simulink model "gm_transmitter"  (R2020b)
settings: Solver=FixedStepDiscrete  StartTime=0.0  StopTime=30  RelTol=1e-3
libraries: dspsigops x3, dspmlti4 x2, hdlmdlgenlib x2, commrandsrc3 x1
settings Model: Creator=wardo  LastModifiedBy=wardo
settings DataIOCC: LimitDataPoints=on  SaveOutput=off  SaveTime=off
settings OptimizationCC: BlockReduction=off  ConditionallyExecuteInputs=off  DefaultParameterBehavior=Inlined  LifeSpan=inf
settings DebuggingCC: AlgebraicLoopMsg=error  InheritedTsInSrcMsg=none  SingleTaskRateTransMsg=error  AllowSymbolicDim=off  StrictBusMsg=ErrorOnBusTreatedAsVector  SFUnexpectedBacktrackingDiag=warning  SFNoUnconditionalDefaultTransitionDiag=warning  SFExecutionAtInitializationDiag=none  ArithmeticOperatorsInVariantConditions=warning
settings HardwareCC: ProdBitPerPointer=32  ProdBitPerSizeT=32  ProdBitPerPtrDiffT=32  ProdLargestAtomicFloat=None  ProdIntDivRoundTo=Undefined  ProdEndianess=Unspecified  ProdWordSize=32  ProdHWDeviceType=ASIC/FPGA->ASIC/FPGA  ProdEqTarget=off
settings SFSimCC: SimUseLocalCustomCode=off  CustomCodeUndefinedFunction=UseInterfaceOnly
settings RTWCC: RTWUseLocalCustomCode=off
settings CodeAppCC: StateflowObjectComments=on
settings GRTTargetCC: TargetLangStandard=C89/C90 (ANSI)
settings ConfigComp: CovScope=ReferencedModels  CovMetricSettings=dw  CovSaveCumulativeToWorkspaceVar=on  CovSaveSingleToWorkspaceVar=on  CovExternalEMLEnable=off  CovSFcnEnable=off

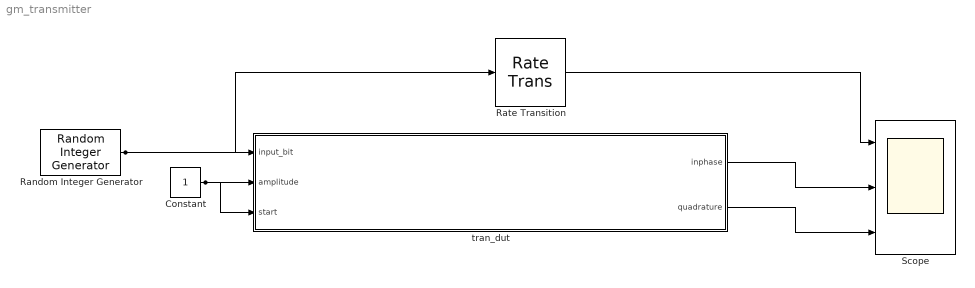
== system gm_transmitter ==
  Constant : Constant  OutDataTypeStr=uint8  SampleTime=-1
  Random Integer Generator : commrandsrc3/Random Integer Generator  SetSize=2  SeedSource=Auto  Seed=0  SampleTime=1  SamplesPerFrame=1  OutputDataType=boolean  SimulateUsing=Code generation
  Rate Transition : RateTransition
  Scope : Scope  NumInputPorts=3
  tran_dut : Subsystem
  wires:
  Rate Transition/1 -> Scope/1
  Constant/1 -> tran_dut/2(amplitude), tran_dut/3(start)
  tran_dut/1(inphase) -> Scope/2
  tran_dut/2(quadrature) -> Scope/3
  Random Integer Generator/1 -> tran_dut/1(input_bit), Rate Transition/1

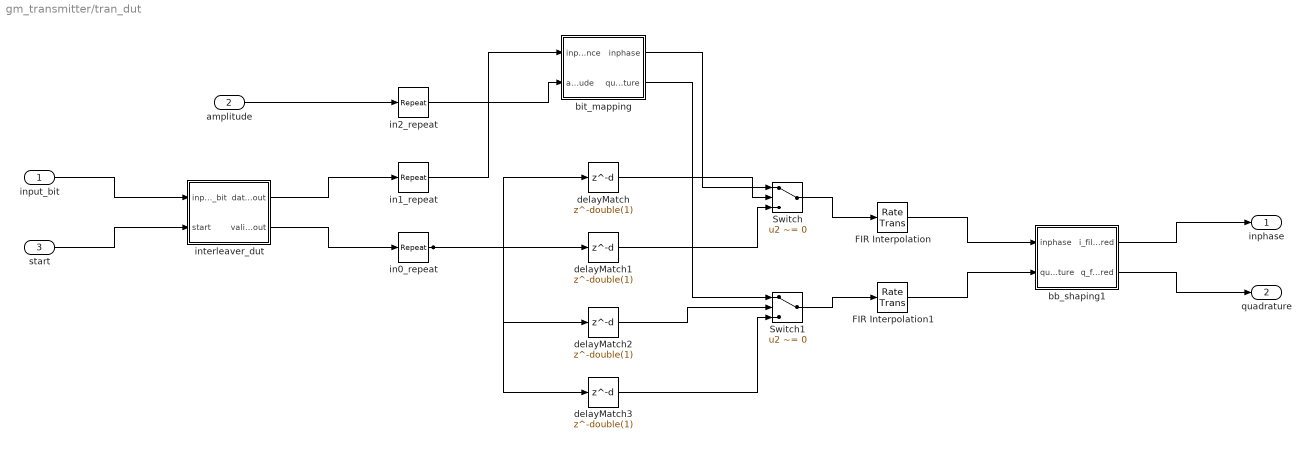
== system gm_transmitter/tran_dut ==
  input_bit : Inport  OutDataTypeStr=boolean  PortDimensions=1  SampleTime=1
  amplitude : Inport  Port=2  OutDataTypeStr=uint8  PortDimensions=1  SampleTime=1
  start : Inport  Port=3  OutDataTypeStr=uint8  PortDimensions=1  SampleTime=1
  FIR Interpolation : RateTransition  OutPortSampleTimeOpt=Multiple of input port sample time  OutPortSampleTimeMultiple=8
  FIR Interpolation1 : RateTransition  OutPortSampleTimeOpt=Multiple of input port sample time  OutPortSampleTimeMultiple=8
  Switch : Switch  Criteria=u2 ~= 0  Threshold=double(0)  OutDataTypeStr=fixdt(1, 25, 15)  SampleTime=0.125
  Switch1 : Switch  Criteria=u2 ~= 0  Threshold=double(0)  OutDataTypeStr=fixdt(1, 25, 15)  SampleTime=0.125
  bb_shaping1 : Subsystem
  bit_mapping : Subsystem
  delayMatch{,1..3} (4 alike) : Delay  DelayLength=double(1)  InitialCondition=0  SampleTime=0.125
  in0_repeat : dspsigops/Repeat  N=double(8)  RateOptions=Allow multirate processing  ic=0  mode=Unused parameter value
  in1_repeat : dspsigops/Repeat  N=double(8)  RateOptions=Allow multirate processing  ic=0  mode=Unused parameter value
  in2_repeat : dspsigops/Repeat  N=double(8)  RateOptions=Allow multirate processing  ic=0  mode=Unused parameter value
  interleaver_dut : Subsystem
  inphase : Outport  VectorParamsAs1DForOutWhenUnconnected=off
  quadrature : Outport  Port=2  VectorParamsAs1DForOutWhenUnconnected=off
  wires:
  input_bit/1 -> interleaver_dut/1(input_bit)
  amplitude/1 -> in2_repeat/1
  start/1 -> interleaver_dut/2(start)
  bb_shaping1/1(i_filtered) -> inphase/1
  bb_shaping1/2(q_filtered) -> quadrature/1
  interleaver_dut/1(data_out) -> in1_repeat/1
  interleaver_dut/2(valid_out) -> in0_repeat/1
  FIR Interpolation/1 -> bb_shaping1/1(inphase)
  FIR Interpolation1/1 -> bb_shaping1/2(quadrature)
  Switch/1 -> FIR Interpolation/1
  Switch1/1 -> FIR Interpolation1/1
  in0_repeat/1 -> delayMatch3/1, delayMatch2/1, delayMatch1/1, delayMatch/1
  in1_repeat/1 -> bit_mapping/1(input_sequence)
  in2_repeat/1 -> bit_mapping/2(amplitude)
  bit_mapping/1(inphase) -> Switch/1
  bit_mapping/2(quadrature) -> Switch1/1
  delayMatch/1 -> Switch/2
  delayMatch1/1 -> Switch/3
  delayMatch2/1 -> Switch1/2
  delayMatch3/1 -> Switch1/3

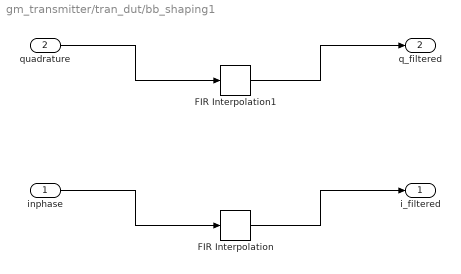
== system gm_transmitter/tran_dut/bb_shaping1 ==
  inphase : Inport  OutDataTypeStr=fixdt(1, 25, 15)  PortDimensions=1  SampleTime=1
  quadrature : Inport  Port=2  OutDataTypeStr=fixdt(1, 25, 15)  PortDimensions=1  SampleTime=1
  FIR Interpolation : dspmlti4/FIR Interpolation  FilterSource=Dialog parameters  PrivateCoeffs=0  h=[-0.00599670410156250,-0.00514221191406250,-0.00289916992187500,0.000442504882812500,0.00431823730468750,0.00794982910156250,0.0104980468750000,0.0112304687500000,0.00967407226562500,0.00578308105468750,0,-0.00680541992187500,-0.0134124755859375,-0.0184326171875000,-0.0205841064453125,-0.0189819335937500,-0.0133361816406250,-0.00410461425781250,0.00752258300781250,0.0196380615234375,0.0300140380859375,0.0363464355468750,0.0367584228515625,0.0301208496093750,0.0164794921875000,-0.00291442871093750,-0.0254821777343750,-0.0476837158203125,-0.0653228759765625,-0.0742187500000000,-0.0707244873046875,-0.0524291992187500,-0.0185852050781250,0.0296783447265625,0.0892028808593750,0.155227661132813,0.221755981445313,0.282333374023438,0.330810546875000,0.362121582031250,0.372940063476563,0.362121582031250,0.330810546875000,0.282333374023438,0.221755981445313,0.155227661132813,0.0892028808593750,0.0296783447265625,-0.0185852050781250,-0.0524291992187500,-0.0707244873046875,-0.0742187500000000,-0.0653228759765625,-0.0476837158203125,-0.0254821777343750,-0.00291442871093750,0.0164794921875000,0.0301208496093750,0.0367584228515625,0.0363464355468750,0.0300140380859375,0.0196380615234375,0.00752258300781250,-0.00410461425781250,-0.0133361816406250,-0.0189819335937500,-0.0205841064453125,-0.0184326171875000,-0.0134124755859375,-0.00680541992187500,0,0.00578308105468750,0.00967407226562500,0.0112304687500000,0.0104980468750000,0.00794982910156250,0.00431823730468750,0.000442504882812500,-0.00289916992187500,-0.00514221191406250,-0.00599670410156250]  L=8  FilterObject=FINTERP  framing=Allow multirate processing  outputBufInitCond=0  roundingMode=Floor  overflowMode=off  firstCoeffMode=Specify word length  firstCoeffWordLength=16  firstCoeffFracLength=15  firstCoeffDataTypeStr=fixdt(1,16)  firstCoeffMin=[]  firstCoeffMax=[]  firstCoeffLastDataTypeStr=fixdt(1,16)  outputDataTypeStr=Inherit: Same as accumulator  outputMin=[]  outputMax=[]  outputLastDataTypeStr=Inherit: Same as accumulator
      settings: SourceProductName=DSP System Toolbox
  FIR Interpolation1 : dspmlti4/FIR Interpolation  FilterSource=Dialog parameters  PrivateCoeffs=0  h=[-0.00599670410156250,-0.00514221191406250,-0.00289916992187500,0.000442504882812500,0.00431823730468750,0.00794982910156250,0.0104980468750000,0.0112304687500000,0.00967407226562500,0.00578308105468750,0,-0.00680541992187500,-0.0134124755859375,-0.0184326171875000,-0.0205841064453125,-0.0189819335937500,-0.0133361816406250,-0.00410461425781250,0.00752258300781250,0.0196380615234375,0.0300140380859375,0.0363464355468750,0.0367584228515625,0.0301208496093750,0.0164794921875000,-0.00291442871093750,-0.0254821777343750,-0.0476837158203125,-0.0653228759765625,-0.0742187500000000,-0.0707244873046875,-0.0524291992187500,-0.0185852050781250,0.0296783447265625,0.0892028808593750,0.155227661132813,0.221755981445313,0.282333374023438,0.330810546875000,0.362121582031250,0.372940063476563,0.362121582031250,0.330810546875000,0.282333374023438,0.221755981445313,0.155227661132813,0.0892028808593750,0.0296783447265625,-0.0185852050781250,-0.0524291992187500,-0.0707244873046875,-0.0742187500000000,-0.0653228759765625,-0.0476837158203125,-0.0254821777343750,-0.00291442871093750,0.0164794921875000,0.0301208496093750,0.0367584228515625,0.0363464355468750,0.0300140380859375,0.0196380615234375,0.00752258300781250,-0.00410461425781250,-0.0133361816406250,-0.0189819335937500,-0.0205841064453125,-0.0184326171875000,-0.0134124755859375,-0.00680541992187500,0,0.00578308105468750,0.00967407226562500,0.0112304687500000,0.0104980468750000,0.00794982910156250,0.00431823730468750,0.000442504882812500,-0.00289916992187500,-0.00514221191406250,-0.00599670410156250]  L=8  FilterObject=FINTERP  framing=Allow multirate processing  outputBufInitCond=0  roundingMode=Floor  overflowMode=off  firstCoeffMode=Specify word length  firstCoeffWordLength=16  firstCoeffFracLength=15  firstCoeffDataTypeStr=fixdt(1,16)  firstCoeffMin=[]  firstCoeffMax=[]  firstCoeffLastDataTypeStr=fixdt(1,16)  outputDataTypeStr=Inherit: Same as accumulator  outputMin=[]  outputMax=[]  outputLastDataTypeStr=Inherit: Same as accumulator
      settings: SourceProductName=DSP System Toolbox
  i_filtered : Outport  VectorParamsAs1DForOutWhenUnconnected=off
  q_filtered : Outport  Port=2  VectorParamsAs1DForOutWhenUnconnected=off
  wires:
  FIR Interpolation/1 -> i_filtered/1
  FIR Interpolation1/1 -> q_filtered/1
  inphase/1 -> FIR Interpolation/1
  quadrature/1 -> FIR Interpolation1/1

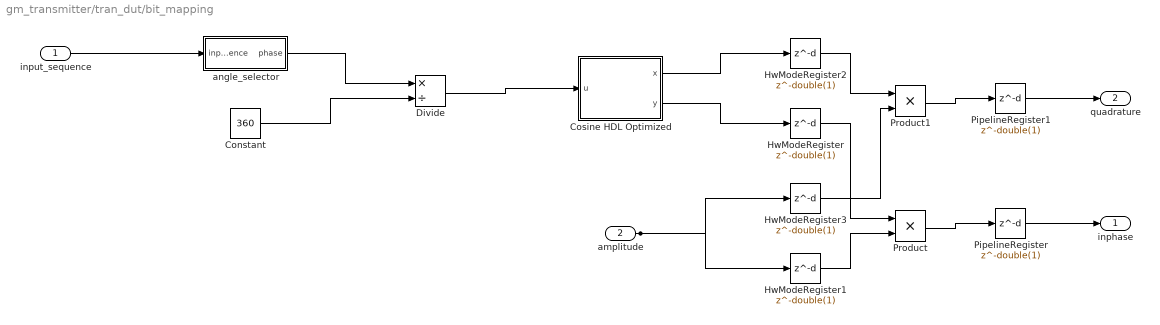
== system gm_transmitter/tran_dut/bit_mapping ==
  input_sequence : Inport  OutDataTypeStr=fixdt(0, 1, 0)  PortDimensions=[1 3]  SampleTime=0.125
  amplitude : Inport  Port=2  OutDataTypeStr=uint8  PortDimensions=1  SampleTime=0.125
  Constant : Constant  Value=360  OutDataTypeStr=fixdt(0, 9, 0)  SampleTime=0.125
  Cosine HDL Optimized : Subsystem  mask(Sine and Cosine HDL optimized block){OutputFormula=sin(2*pi*u) and cos(2*pi*u), NumDataPoints=double(64), TableDataTypeStr=fixdt(1,16,15), SimulateLUTROMDelay=off}
      mask prompts: OutputFormula "Simulink:masks:OutputFormula_MP"; NumDataPoints "HDLShared:hdlshared:CosineHDL_Npts"; TableDataTypeStr "Simulink:blkprm_prompts:TABLE_UNIFIEDDATATYPE"; SimulateLUTROMDelay "HDLShared:hdlshared:CosineHDL_Map2RAM"
      mask help: Sine and Cosine HDL optimized block using quarter wave symmetry, and HDL friendly settings.
      mask Help: helpview([docroot '/hdlcoder/helptargets.map'],'SineAndCosineHDL_Optimized');
      mask TypeOptions OutputFormula: sin(2*pi*u) | cos(2*pi*u) | exp(j*2*pi*u) | sin(2*pi*u) and cos(2*pi*u)
      mask Display:
      | port_label('input',1,'u')
      | port_label('output',1,'sin(2*pi*u)')
      | port_label('output',2,'cos(2*pi*u)')
      | xpos = 0.35;
      | yoffset = 0.5;
      | if ( SimulateLUTROMDelay )
      |   text(xpos,yoffset,'HDL (Z^{-1})','texmode','on')
      | else
      |    text(xpos,yoffset,'HDL')
      | end
  Divide : Product  Inputs=*/  OutDataTypeStr=fixdt(1, 16, 14)  RndMeth=Zero  SaturateOnIntegerOverflow=on  SampleTime=0.125
  HwModeRegister{,1..3} (4 alike) : Delay  DelayLength=double(1)  InitialCondition=0  SampleTime=0.125
  PipelineRegister : Delay  DelayLength=double(1)  InitialCondition=0  SampleTime=0.125
  PipelineRegister1 : Delay  DelayLength=double(1)  InitialCondition=0  SampleTime=0.125
  Product : Product  Inputs=**  OutDataTypeStr=fixdt(1, 25, 15)  SampleTime=0.125
  Product1 : Product  Inputs=**  OutDataTypeStr=fixdt(1, 25, 15)  SampleTime=0.125
  angle_selector : Subsystem
  inphase : Outport  VectorParamsAs1DForOutWhenUnconnected=off
  quadrature : Outport  Port=2  VectorParamsAs1DForOutWhenUnconnected=off
  wires:
  Constant/1 -> Divide/2
  Cosine HDL Optimized/1(x) -> HwModeRegister2/1
  Cosine HDL Optimized/2(y) -> HwModeRegister/1
  Divide/1 -> Cosine HDL Optimized/1(u)
  PipelineRegister/1 -> inphase/1
  PipelineRegister1/1 -> quadrature/1
  angle_selector/1(phase) -> Divide/1
  input_sequence/1 -> angle_selector/1(input_sequence)
  amplitude/1 -> HwModeRegister1/1, HwModeRegister3/1
  Product/1 -> PipelineRegister/1
  HwModeRegister/1 -> Product/1
  HwModeRegister1/1 -> Product/2
  Product1/1 -> PipelineRegister1/1
  HwModeRegister2/1 -> Product1/1
  HwModeRegister3/1 -> Product1/2

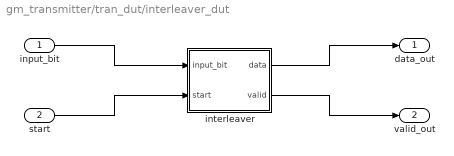
== system gm_transmitter/tran_dut/interleaver_dut ==
  input_bit : Inport  OutDataTypeStr=boolean  PortDimensions=1  SampleTime=1
  start : Inport  Port=2  OutDataTypeStr=uint8  PortDimensions=1  SampleTime=1
  interleaver : Subsystem
  data_out : Outport  VectorParamsAs1DForOutWhenUnconnected=off
  valid_out : Outport  Port=2  VectorParamsAs1DForOutWhenUnconnected=off
  wires:
  interleaver/1(data) -> data_out/1
  interleaver/2(valid) -> valid_out/1
  input_bit/1 -> interleaver/1(input_bit)
  start/1 -> interleaver/2(start)

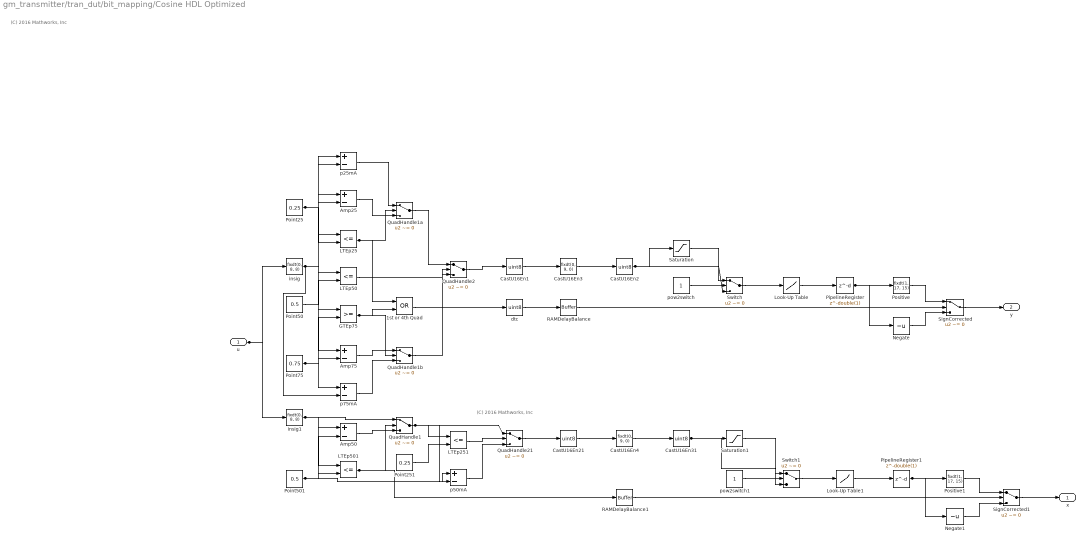
== system gm_transmitter/tran_dut/bit_mapping/Cosine HDL Optimized ==
  note: (C) 2016 Mathworks, Inc
  note: (C) 2016 Mathworks, Inc
  u : Inport  OutDataTypeStr=fixdt(1, 16, 14)  SampleTime=0.125
  1st or 4th Quad : Logic  Operator=OR  AllPortsSameDT=off  OutDataTypeStr=boolean  SampleTime=0.125
  Amp25 : Sum  Inputs=+-  AccumDataTypeStr=fixdt(1, 18, 17)  OutDataTypeStr=fixdt(1, 18, 17)  SampleTime=0.125
  Amp50 : Sum  Inputs=+-  AccumDataTypeStr=fixdt(1, 18, 17)  OutDataTypeStr=fixdt(1, 18, 17)  SampleTime=0.125
  Amp75 : Sum  Inputs=+-  AccumDataTypeStr=fixdt(1, 18, 17)  OutDataTypeStr=fixdt(1, 18, 17)  SampleTime=0.125
  CastU16En1 : DataTypeConversion  OutDataTypeStr=uint8  ConvertRealWorld=Stored Integer (SI)  SampleTime=0.125
  CastU16En2 : DataTypeConversion  OutDataTypeStr=uint8  ConvertRealWorld=Stored Integer (SI)  SampleTime=0.125  SaturateOnIntegerOverflow=on
  CastU16En21 : DataTypeConversion  OutDataTypeStr=uint8  ConvertRealWorld=Stored Integer (SI)  SampleTime=0.125
  CastU16En3 : DataTypeConversion  OutDataTypeStr=fixdt(0, 9, 0)  SampleTime=0.125
  CastU16En31 : DataTypeConversion  OutDataTypeStr=uint8  ConvertRealWorld=Stored Integer (SI)  SampleTime=0.125  SaturateOnIntegerOverflow=on
  CastU16En4 : DataTypeConversion  OutDataTypeStr=fixdt(0, 9, 0)  SampleTime=0.125
  GTEp75 : RelationalOperator  OutDataTypeStr=boolean  SampleTime=0.125  RndMeth=Nearest
  LTEp{25,50,251,501} (4 alike) : RelationalOperator  Operator=<=  OutDataTypeStr=boolean  SampleTime=0.125  RndMeth=Nearest
  Look-Up Table : Lookup_n-D  NumberOfTableDimensions=1  BreakpointsForDimension1="fi(\"numerictype\",numerictype(0,8,0),\"fimath\",fimath(\"RoundingMethod\", \"Floor\",\"OverflowAction\", \"Wrap\",\"ProductMode\",\"FullPrecision\",\"SumMode\",\"FullPrecision\"),\"Value\",\"[0 1 2 3 4 5 6 7 8 9 10 11 12 13 14 15 16 17 18 19 20 21 22 23 24 25 26 27 28 29 30 31 32 33 34 35 36 37 38 39 40 41 42 43 44 45 46 47 48 49 50 51 52 53 54 55 56 57 58 59 60 61 62 63]\")"  Table="reshape(fi(\"numerictype\",numerictype(1,17,15),\"fimath\",fimath(\"RoundingMethod\", \"Floor\",\"OverflowAction\", \"Wrap\",\"ProductMode\",\"FullPrecision\",\"SumMode\",\"FullPrecision\"),\"Value\",\"[0;0.024932861328125;0.049835205078125;0.074737548828125;0.099578857421875;0.12432861328125;0.1490478515625;0.17364501953125;0.198150634765625;0.2225341796875;0.24676513671875;0.270843505859375;0.294769287109375;0.3184814453125;0.342010498046875;0.365325927734375;0.388427734375;0.411285400390625;0.43389892578125;0.456207275390625;0.478240966796875;0.5;0.52142333984375;0.54254150390625;0.563323974609375;0.583740234375;0.603790283203125;0.623504638671875;0.642791748046875;0.66168212890625;0.68017578125;0.6982421875;0.71588134765625;0.733062744140625;0.749786376953125;0.76605224609375;0.781829833984375;0.797119140625;0.81195068359375;0.82623291015625;0.84002685546875;0.853302001953125;0.86602783203125;0.87823486328125;0.889862060546875;0.900970458984375;0.9114990234375;0.921478271484375;0.930877685546875;0.939697265625;0.94793701171875;0.95556640625;0.962615966796875;0.969085693359375;0.97491455078125;0.98016357421875;0.98480224609375;0.98883056640625;0.99224853515625;0.995025634765625;0.9971923828125;0.998748779296875;0.99969482421875;1]\"), [1  64])"  InterpMethod=Flat  ExtrapMethod=Clip  DiagnosticForOutOfRangeInput=Error  SampleTime=0.125  OutDataTypeStr=fixdt(1, 17, 15)  InputSameDT=on
  Look-Up Table1 : Lookup_n-D  NumberOfTableDimensions=1  BreakpointsForDimension1="fi(\"numerictype\",numerictype(0,8,0),\"fimath\",fimath(\"RoundingMethod\", \"Floor\",\"OverflowAction\", \"Wrap\",\"ProductMode\",\"FullPrecision\",\"SumMode\",\"FullPrecision\"),\"Value\",\"[0 1 2 3 4 5 6 7 8 9 10 11 12 13 14 15 16 17 18 19 20 21 22 23 24 25 26 27 28 29 30 31 32 33 34 35 36 37 38 39 40 41 42 43 44 45 46 47 48 49 50 51 52 53 54 55 56 57 58 59 60 61 62 63]\")"  Table="reshape(fi(\"numerictype\",numerictype(1,17,15),\"fimath\",fimath(\"RoundingMethod\", \"Floor\",\"OverflowAction\", \"Wrap\",\"ProductMode\",\"FullPrecision\",\"SumMode\",\"FullPrecision\"),\"Value\",\"[0;0.024932861328125;0.049835205078125;0.074737548828125;0.099578857421875;0.12432861328125;0.1490478515625;0.17364501953125;0.198150634765625;0.2225341796875;0.24676513671875;0.270843505859375;0.294769287109375;0.3184814453125;0.342010498046875;0.365325927734375;0.388427734375;0.411285400390625;0.43389892578125;0.456207275390625;0.478240966796875;0.5;0.52142333984375;0.54254150390625;0.563323974609375;0.583740234375;0.603790283203125;0.623504638671875;0.642791748046875;0.66168212890625;0.68017578125;0.6982421875;0.71588134765625;0.733062744140625;0.749786376953125;0.76605224609375;0.781829833984375;0.797119140625;0.81195068359375;0.82623291015625;0.84002685546875;0.853302001953125;0.86602783203125;0.87823486328125;0.889862060546875;0.900970458984375;0.9114990234375;0.921478271484375;0.930877685546875;0.939697265625;0.94793701171875;0.95556640625;0.962615966796875;0.969085693359375;0.97491455078125;0.98016357421875;0.98480224609375;0.98883056640625;0.99224853515625;0.995025634765625;0.9971923828125;0.998748779296875;0.99969482421875;1]\"), [1  64])"  InterpMethod=Flat  ExtrapMethod=Clip  DiagnosticForOutOfRangeInput=Error  SampleTime=0.125  OutDataTypeStr=fixdt(1, 17, 15)  InputSameDT=on
  Negate : UnaryMinus  SampleTime=0.125
  Negate1 : UnaryMinus  SampleTime=0.125
  PipelineRegister : Delay  DelayLength=double(1)  InitialCondition=0  SampleTime=0.125
  PipelineRegister1 : Delay  DelayLength=double(1)  InitialCondition=0  SampleTime=0.125
  Point25 : Constant  Value=0.25  OutDataTypeStr=fixdt(0, 17, 17)  SampleTime=0.125
  Point251 : Constant  Value=0.25  OutDataTypeStr=fixdt(0, 17, 17)  SampleTime=0.125
  Point50 : Constant  Value=0.5  OutDataTypeStr=fixdt(0, 17, 17)  SampleTime=0.125
  Point501 : Constant  Value=0.5  OutDataTypeStr=fixdt(0, 17, 17)  SampleTime=0.125
  Point75 : Constant  Value=0.75  OutDataTypeStr=fixdt(0, 17, 17)  SampleTime=0.125
  Positive : DataTypeConversion  OutDataTypeStr=fixdt(1, 17, 15)  SampleTime=0.125
  Positive1 : DataTypeConversion  OutDataTypeStr=fixdt(1, 17, 15)  SampleTime=0.125
  QuadHandle1 : Switch  Criteria=u2 ~= 0  Threshold=double(0)  OutDataTypeStr=fixdt(1, 18, 17)  SampleTime=0.125
  QuadHandle1a : Switch  Criteria=u2 ~= 0  Threshold=double(0)  OutDataTypeStr=fixdt(1, 18, 17)  SampleTime=0.125
  QuadHandle1b : Switch  Criteria=u2 ~= 0  Threshold=double(0)  OutDataTypeStr=fixdt(1, 18, 17)  SampleTime=0.125
  QuadHandle2 : Switch  Criteria=u2 ~= 0  Threshold=double(0)  OutDataTypeStr=fixdt(0, 8, 8)  SampleTime=0.125  SaturateOnIntegerOverflow=on
  QuadHandle21 : Switch  Criteria=u2 ~= 0  Threshold=double(0)  OutDataTypeStr=fixdt(0, 8, 8)  SampleTime=0.125
  RAMDelayBalance : hdlmdlgenlib/Buffer
      settings: SourceProductBaseCode=SL
  RAMDelayBalance1 : hdlmdlgenlib/Buffer
      settings: SourceProductBaseCode=SL
  Saturation : Saturate  UpperLimit="fi(0,0,8,0,\"hex\",\"3f\")"  LowerLimit="fi(0,0,8,0,\"hex\",\"00\")"  SampleTime=0.125  OutDataTypeStr=uint8
  Saturation1 : Saturate  UpperLimit="fi(0,0,8,0,\"hex\",\"3f\")"  LowerLimit="fi(0,0,8,0,\"hex\",\"00\")"  SampleTime=0.125  OutDataTypeStr=uint8
  SignCorrected : Switch  Criteria=u2 ~= 0  Threshold=double(0)  OutDataTypeStr=fixdt(1, 17, 15)  SampleTime=0.125
  SignCorrected1 : Switch  Criteria=u2 ~= 0  Threshold=double(0)  OutDataTypeStr=fixdt(1, 17, 15)  SampleTime=0.125
  Switch : Switch  Criteria=u2 ~= 0  Threshold=double(0)  OutDataTypeStr=uint8  SampleTime=0.125
  Switch1 : Switch  Criteria=u2 ~= 0  Threshold=double(0)  OutDataTypeStr=uint8  SampleTime=0.125
  dtc : DataTypeConversion  OutDataTypeStr=uint8  SampleTime=0.125
  insig : DataTypeConversion  OutDataTypeStr=fixdt(0, 8, 8)  SampleTime=0.125
  insig1 : DataTypeConversion  OutDataTypeStr=fixdt(0, 8, 8)  SampleTime=0.125
  p25mA : Sum  Inputs=+-  AccumDataTypeStr=fixdt(1, 18, 17)  OutDataTypeStr=fixdt(1, 18, 17)  SampleTime=0.125
  p50mA : Sum  Inputs=+-  AccumDataTypeStr=fixdt(1, 19, 17)  OutDataTypeStr=fixdt(1, 19, 17)  SampleTime=0.125
  p75mA : Sum  Inputs=+-  AccumDataTypeStr=fixdt(1, 18, 17)  OutDataTypeStr=fixdt(1, 18, 17)  SampleTime=0.125
  pow2switch : Constant  OutDataTypeStr=boolean  SampleTime=0.125
  pow2switch1 : Constant  OutDataTypeStr=boolean  SampleTime=0.125
  x : Outport
  y : Outport  Port=2
  wires:
  dtc/1 -> RAMDelayBalance/1
  Amp25/1 -> QuadHandle1a/3
  Amp75/1 -> QuadHandle1b/1
  CastU16En1/1 -> CastU16En3/1
  CastU16En2/1 -> Switch/3, Saturation/1
  CastU16En3/1 -> CastU16En2/1
  GTEp75/1 -> QuadHandle1b/2, 1st or 4th Quad/2
  LTEp25/1 -> QuadHandle1a/2, 1st or 4th Quad/1
  LTEp50/1 -> QuadHandle2/2
  PipelineRegister/1 -> Positive/1, Negate/1
  Negate/1 -> SignCorrected/3
  Point25/1 -> p25mA/1, LTEp25/2, Amp25/2
  Point50/1 -> LTEp50/2
  Point75/1 -> p75mA/1, GTEp75/2, Amp75/2
  Positive/1 -> SignCorrected/1
  QuadHandle1a/1 -> QuadHandle2/1
  QuadHandle1b/1 -> QuadHandle2/3
  QuadHandle2/1 -> CastU16En1/1
  Saturation/1 -> Switch/1
  SignCorrected/1 -> y/1
  Switch/1 -> Look-Up Table/1
  insig/1 -> p75mA/2, p25mA/2, LTEp50/1, LTEp25/1, GTEp75/1, Amp75/1, Amp25/1
  p25mA/1 -> QuadHandle1a/1
  p75mA/1 -> QuadHandle1b/3
  pow2switch/1 -> Switch/2
  Amp50/1 -> QuadHandle1/3
  CastU16En21/1 -> CastU16En4/1
  CastU16En31/1 -> Switch1/3, Saturation1/1
  CastU16En4/1 -> CastU16En31/1
  LTEp251/1 -> QuadHandle21/2
  LTEp501/1 -> QuadHandle1/2, RAMDelayBalance1/1
  PipelineRegister1/1 -> Positive1/1, Negate1/1
  Negate1/1 -> SignCorrected1/3
  Point251/1 -> LTEp251/2
  Point501/1 -> p50mA/1, LTEp501/2, Amp50/2
  Positive1/1 -> SignCorrected1/1
  QuadHandle1/1 -> p50mA/2, QuadHandle21/1, LTEp251/1
  QuadHandle21/1 -> CastU16En21/1
  Saturation1/1 -> Switch1/1
  SignCorrected1/1 -> x/1
  Switch1/1 -> Look-Up Table1/1
  insig1/1 -> QuadHandle1/1, LTEp501/1, Amp50/1
  p50mA/1 -> QuadHandle21/3
  pow2switch1/1 -> Switch1/2
  1st or 4th Quad/1 -> dtc/1
  RAMDelayBalance1/1 -> SignCorrected1/2
  RAMDelayBalance/1 -> SignCorrected/2
  u/1 -> insig1/1, insig/1
  Look-Up Table/1 -> PipelineRegister/1
  Look-Up Table1/1 -> PipelineRegister1/1

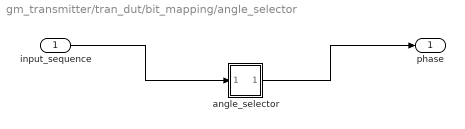
== system gm_transmitter/tran_dut/bit_mapping/angle_selector ==
  input_sequence : Inport  OutDataTypeStr=fixdt(0, 1, 0)  PortDimensions=[1 3]  SampleTime=0.125
  angle_selector : MATLAB Function  TreatAsAtomicUnit=on
  phase : Outport  VectorParamsAs1DForOutWhenUnconnected=off
  wires:
  angle_selector/1(phase) -> phase/1
  input_sequence/1 -> angle_selector/1(input_sequence)

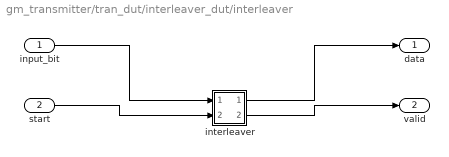
== system gm_transmitter/tran_dut/interleaver_dut/interleaver ==
  input_bit : Inport  OutDataTypeStr=boolean  PortDimensions=1  SampleTime=1
  start : Inport  Port=2  OutDataTypeStr=uint8  PortDimensions=1  SampleTime=1
  interleaver : MATLAB Function  TreatAsAtomicUnit=on
  data : Outport  VectorParamsAs1DForOutWhenUnconnected=off
  valid : Outport  Port=2
  wires:
  interleaver/1(data) -> data/1
  interleaver/2(valid) -> valid/1
  input_bit/1 -> interleaver/1(input_bit)
  start/1 -> interleaver/2(start)

== matlab function gm_transmitter/tran_dut/bit_mapping/angle_selector/angle_selector ==
  settings: fimath=fimath('RoundingMethod', 'Floor','OverflowAction', 'Wrap','ProductMode', 'FullPrecision', 'SumMode', 'FullPrecision')
  data: input_sequence input; phase output
function phase = phase_selector(input_sequence)
%#codegen
% Receives a bit sequence and returns the angle in radians of the
% corresponding 8-psk constellation symbol. Gray encoding is used as stated
% in the DVB-S2 standard.
    tmp = 0; % Start at phase 0
    if(input_sequence(1)==0 && input_sequence(2)==0 && input_sequence(3)==1)
        tmp=0;
    elseif(input_sequence(1)==0 && input_sequence(2)==0 && input_sequence(3)==0)
        tmp=45;
    elseif(input_sequence(1)==1 && input_sequence(2)==0 && input_sequence(3)==0)
        tmp=90;
    elseif(input_sequence(1)==1 && input_sequence(2)==1 && input_sequence(3)==0)
        tmp=135;
    elseif(input_sequence(1)==0 && input_sequence(2)==1 && input_sequence(3)==0)
        tmp=180;
    elseif(input_sequence(1)==0 && input_sequence(2)==1 && input_sequence(3)==1)
        tmp=225;
    elseif(input_sequence(1)==1 && input_sequence(2)==1 && input_sequence(3)==1)
        tmp=270;
    elseif(input_sequence(1)==1 && input_sequence(2)==0 && input_sequence(3)==1)
        tmp=315;
    end
    % 9 bits necessary to represent 360 degrees.
    phase = fi(tmp, 0, 23, 14, hdlfimath);

== matlab function gm_transmitter/tran_dut/interleaver_dut/interleaver/interleaver ==
  settings: fimath=fimath('RoundingMethod', 'Floor','OverflowAction', 'Wrap','ProductMode', 'FullPrecision', 'SumMode', 'FullPrecision')
  data: input_bit input; data output; start input; valid output
function [data, valid] = fsm_interleaver(input_bit, start)
%#codegen

rows           = 4;
columns        = 3;
state_iddle    = 0;
state_writting = 1;
state_reading  = 2;

persistent moore_state_reg;
if isempty(moore_state_reg)
    moore_state_reg = fi(0, 0, 2, 0);   
end

persistent counter;
if isempty(counter)
    counter = fi(1, 0, 16, 0);
end

persistent column;
if isempty(column)
    column = fi(1, 0, 8, 0);   
end

persistent buffer;
if isempty(buffer)
    buffer = fi(zeros(rows, columns), 0, 1, 0);
end

switch (moore_state_reg)
    
    case state_iddle
        counter = fi(1, 0, 16, 0);   
        column  = fi(1, 0, 8, 0);   
        buffer  = fi(zeros(rows, columns), 0, 1, 0);
        valid   = false;
        data    = fi([0 0 0], 0, 1, 0);
        if (~start)
            moore_state_reg(1) = state_iddle;
        else
            moore_state_reg(1) = state_writting;
            % Write first bit at the bottom-rightest bit of the buffer
            buffer(rows - counter + 1, columns - column + 1) = input_bit;
            counter = fi(counter + 1, 0, 16, 0);
        end
        
    case state_writting
        buffer(rows - counter + 1, columns - column + 1) = input_bit;
        counter = fi(counter + 1, 0, 16, 0);
        if counter > rows
            counter = fi(1, 0, 16, 0);
            column  = fi(column + 1, 0, 8, 0);
            if (column > columns)
                moore_state_reg(1) = state_reading;
                counter = fi(1, 0, 16, 0);   
                column  = fi(1, 0, 8, 0);   
                valid   = true;
                data    = buffer(counter, :);
                counter = fi(counter + 1, 0, 16, 0);
            else
                data    = fi([0 0 0], 0, 1, 0);
                valid   = false;
            end
        else
            valid   = false;
            data    = fi([0 0 0], 0, 1, 0);
        end
    case state_reading
        data = buffer(counter, :);
        counter = fi(counter + 1, 0, 16, 0);
        if counter > rows
            moore_state_reg(1) = state_iddle;
        end
        valid = true;
    otherwise
        valid = false;
        data  = fi([0 0 0], 0, 1, 0);      
end
